simulink model "ex3_sim2"  (R2018a)
settings: Solver=ode45  StartTime=0.0  StopTime=5  MaxStep=0.01  RelTol=1e-3  EnableMultiTasking=on
undefined symbols (not defined in the file): Ar, d0, denH, DiscIntNeverNeededParam, Kd, Ki, km, Kp, numH, Tm, Ts, wr
settings Model: Creator=antonello  LastModifiedBy=riccardo
settings DataIOCC: LimitDataPoints=on  SaveFormat=Array
settings OptimizationCC: LifeSpan=inf
settings DebuggingCC: SolverPrmCheckMsg=warning  SFUnexpectedBacktrackingDiag=warning  SFNoUnconditionalDefaultTransitionDiag=warning  SFExecutionAtInitializationDiag=none
settings HardwareCC: ProdBitPerPointer=32  ProdBitPerSizeT=32  ProdBitPerPtrDiffT=32  ProdLargestAtomicFloat=None  ProdIntDivRoundTo=Undefined  ProdEndianess=Unspecified  ProdWordSize=32  ProdHWDeviceType=32-bit Generic
settings ModelReferenceCC: PropagateSignalLabelsOutOfModel=off
settings CodeAppCC: StateflowObjectComments=on
settings GRTTargetCC: TargetLangStandard=C89/C90 (ANSI)  GeneratePreprocessorConditionals=Disable all
settings ConfigComp: CovMetricSettings=dw  CovHtmlReporting=on  CovSaveCumulativeToWorkspaceVar=on  CovSaveSingleToWorkspaceVar=on  CovExternalEMLEnable=off  CovSFcnEnable=off

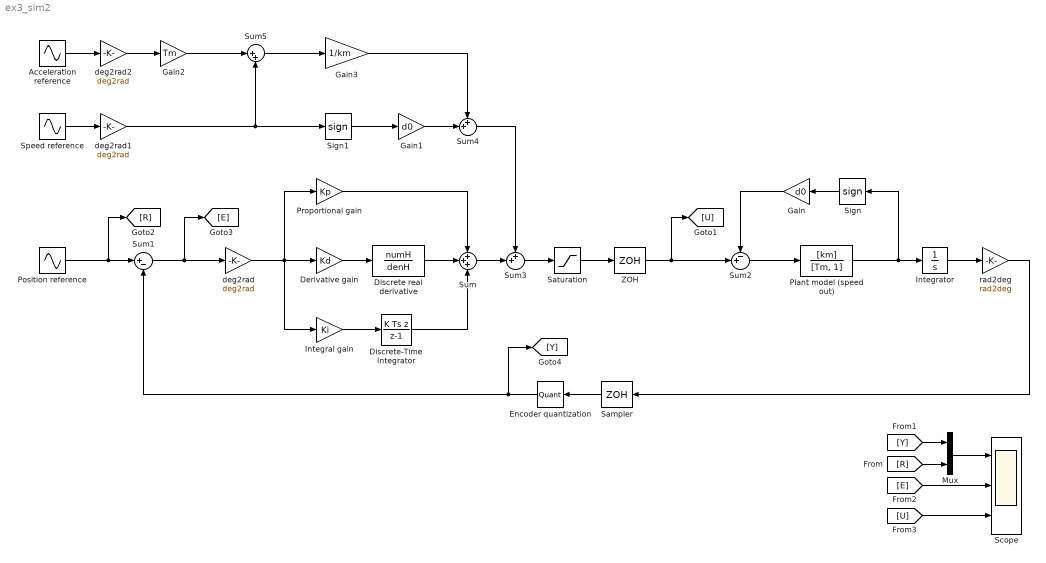
== system ex3_sim2 ==
  Acceleration reference : Sin  Amplitude=-Ar*wr^2  Frequency=wr  SampleTime=0
  Derivative gain : Gain  Gain=Kd
  Discrete real derivative : DiscreteTransferFcn  Numerator=numH  Denominator=denH  SampleTime=Ts
  Discrete-Time Integrator : DiscreteIntegrator  IntegratorMethod=Integration: Backward Euler  SampleTime=Ts  ICPrevOutput=DiscIntNeverNeededParam  ICPrevScaledInput=DiscIntNeverNeededParam
  Encoder quantization : Quantizer  QuantizationInterval=enc_pulse2deg
  Gain : Gain  Gain=d0
  Gain1 : Gain  Gain=d0
  Gain2 : Gain  Gain=Tm
  Gain3 : Gain  Gain=1/km
  Integral gain : Gain  Gain=Ki
  Integrator : Integrator
  Mux : Mux  Inputs=2
  Plant model (speed out) : TransferFcn  Numerator=[km]  Denominator=[Tm, 1]
  Position reference : Sin  Amplitude=Ar  Frequency=wr  SampleTime=0
  Proportional gain : Gain  Gain=Kp
  Sampler : ZeroOrderHold  SampleTime=Ts
  Saturation : Saturate  UpperLimit=10  LowerLimit=-10
  Scope : Scope  NumInputPorts=3
  Sign : Signum  ZeroCross=off
  Sign1 : Signum  ZeroCross=off
  Speed reference : Sin  Amplitude=Ar*wr  Frequency=wr  Phase=pi/2  SampleTime=0
  Sum : Sum  Inputs=+++
  Sum1 : Sum  Inputs=|+-
  Sum2 : Sum  Inputs=-+|
  Sum3 : Sum  Inputs=++|
  Sum4 : Sum  Inputs=++|
  Sum5 : Sum  Inputs=|++
  ZOH : ZeroOrderHold  SampleTime=Ts
  deg2rad : Gain  Gain=deg2rad
  deg2rad1 : Gain  Gain=deg2rad
  deg2rad2 : Gain  Gain=deg2rad
  rad2deg : Gain  Gain=rad2deg
  wires:
  Derivative gain/1 -> Discrete real derivative/1
  Integral gain/1 -> Discrete-Time Integrator/1
  Proportional gain/1 -> Sum/1
  Sum1/1 -> [E], deg2rad/1
  Plant model (speed out)/1 -> Sign/1, Integrator/1
  ZOH/1 -> Sum2/2, [U]
  Position reference/1 -> [R], Sum1/1
  Discrete real derivative/1 -> Sum/2
  Discrete-Time Integrator/1 -> Sum/3
  [Y] -> Mux/1
  [R] -> Mux/2
  Mux/1 -> Scope/1
  [E] -> Scope/2
  [U] -> Scope/3
  rad2deg/1 -> Sampler/1
  deg2rad/1 -> Integral gain/1, Derivative gain/1, Proportional gain/1
  Sampler/1 -> Encoder quantization/1
  Encoder quantization/1 -> Sum1/2, [Y]
  Sum2/1 -> Plant model (speed out)/1
  Integrator/1 -> rad2deg/1
  Sign/1 -> Gain/1
  Sum3/1 -> Saturation/1
  Sum/1 -> Sum3/2
  Speed reference/1 -> deg2rad1/1
  Saturation/1 -> ZOH/1
  Sign1/1 -> Gain1/1
  Gain2/1 -> Sum5/1
  Acceleration reference/1 -> deg2rad2/1
  Gain3/1 -> Sum4/1
  Gain1/1 -> Sum4/2
  Sum4/1 -> Sum3/1
  Gain/1 -> Sum2/1
  deg2rad1/1 -> Sign1/1, Sum5/2
  deg2rad2/1 -> Gain2/1
  Sum5/1 -> Gain3/1
